simulink model "digitaler_zr"  (R2022b)
settings: Solver=ode45  StartTime=0.0  StopTime=tsim  FixedStep=0.00025  RelTol=1e-3  EnableMultiTasking=on
values from neighbouring files (symbols this model uses):
  A = double(subs(A))    [init1.m]
  B = double(subs(B))    [init1.m]
  C = double(subs(C))    [init1.m]
  q1z = double(subs(q1z))    [init1.m]
  q1zb = double(subs(q1zb))    [init1.m]
  q1zbin = double(subs(q1zbin))    [init1.m]
  R = double(subs(R))    [init1.m]
  Rb = double(subs(Rb))    [init1.m]
  Rbin = double(subs(Rbin))    [init1.m]
  T = 0.5e-3    (= 0.0005)    [init1.m]
  TR = double(subs(TR))    [init1.m]
  tstep = 0.05    [init1.m]
settings Model: Creator=axel  LastModifiedBy=kraie
settings SolverCC: AlgebraicLoopSolver=TrustRegion
settings DataIOCC: LimitDataPoints=on  SaveFormat=Array  SignalLoggingSaveFormat=ModelDataLogs  ReturnWorkspaceOutputs=off
settings OptimizationCC: ExpressionDepthLimit=2147483647  InitFltsAndDblsToZero=on  LifeSpan=inf
settings DebuggingCC: SaveWithParameterizedLinksMsg=none  UnderspecifiedInitializationDetection=Classic  MergeDetectMultiDrivingBlocksExec=none  SignalResolutionControl=TryResolveAllWithWarning  SolverPrmCheckMsg=warning  MultiTaskDSMMsg=warning  MultiTaskCondExecSysMsg=none  FcnCallInpInsideContextMsg=warning  UnconnectedInputMsg=warning  UnconnectedOutputMsg=warning  UnconnectedLineMsg=warning  StateNameClashWarn=warning  SFUnexpectedBacktrackingDiag=warning  SFNoUnconditionalDefaultTransitionDiag=warning  SFMachineParentedDataDiag=warning  ArithmeticOperatorsInVariantConditions=warning
settings HardwareCC: ProdBitPerPointer=32  ProdBitPerSizeT=32  ProdBitPerPtrDiffT=32  ProdLargestAtomicFloat=None  ProdIntDivRoundTo=Undefined  ProdEndianess=Unspecified  ProdWordSize=32  ProdHWDeviceType=32-bit Generic
settings ModelReferenceCC: EnableRefExpFcnMdlSchedulingChecks=on  PropagateSignalLabelsOutOfModel=off
settings SFSimCC: SimUseLocalCustomCode=off  CustomCodeUndefinedFunction=UseInterfaceOnly
settings RTWCC: RTWUseLocalCustomCode=off
settings CodeAppCC: StateflowObjectComments=on
settings GRTTargetCC: TargetFcnLib=ansi_tfl_tmw.mat  TargetLangStandard=C89/C90 (ANSI)  CombineOutputUpdateFcns=off  GRTInterface=on
settings ConfigComp: CovMetricSettings=dw  CovSaveCumulativeToWorkspaceVar=on  CovSaveSingleToWorkspaceVar=on  CovExternalEMLEnable=off

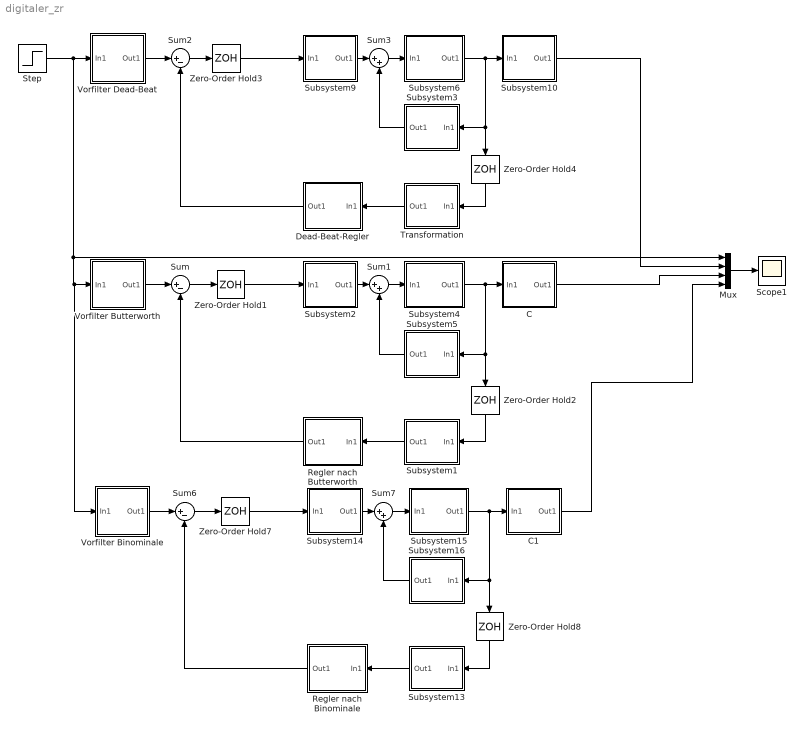
== system digitaler_zr ==
  C : Subsystem
      mask Display: disp('C')
  C1 : Subsystem
      mask Display: disp('C')
  Dead-Beat-Regler : Subsystem
      mask Display: disp('R\nDead-Beat')
  Mux : Mux
  Regler nach Binominale : Subsystem
      mask Display: disp('Rb\nButterworth')
  Regler nach Butterworth : Subsystem
      mask Display: disp('Rb\nButterworth')
  Scope1 : Scope
  Step : Step  Time=tstep  SampleTime=0
  Subsystem1 : Subsystem
      mask Display: disp('TR')
  Subsystem10 : Subsystem
      mask Display: disp('C')
  Subsystem13 : Subsystem
      mask Display: disp('TR')
  Subsystem14 : Subsystem
      mask Display: disp('B')
  Subsystem15 : Subsystem
      mask Display: plot([0.3 0.35 0.4 0.45 0.55 0.6 0.65 0.7], [0.3 0.21 0.2 0.3 0.7 0.8 0.79 0.7]);
  Subsystem16 : Subsystem
      mask Display: disp('A')
  Subsystem2 : Subsystem
      mask Display: disp('B')
  Subsystem3 : Subsystem
      mask Display: disp('A')
  Subsystem4 : Subsystem
      mask Display: plot([0.3 0.35 0.4 0.45 0.55 0.6 0.65 0.7], [0.3 0.21 0.2 0.3 0.7 0.8 0.79 0.7]);
  Subsystem5 : Subsystem
      mask Display: disp('A')
  Subsystem6 : Subsystem
      mask Display: plot([0.3 0.35 0.4 0.45 0.55 0.6 0.65 0.7], [0.3 0.21 0.2 0.3 0.7 0.8 0.79 0.7]);
  Subsystem9 : Subsystem
      mask Display: disp('B')
  Sum : Sum  Inputs=|+-
  Sum1 : Sum  Inputs=|++
  Sum2 : Sum  Inputs=|+-
  Sum3 : Sum  Inputs=|++
  Sum6 : Sum  Inputs=|+-
  Sum7 : Sum  Inputs=|++
  Transformation : Subsystem
      mask Display: disp('TR')
  Vorfilter Binominale : Subsystem
      mask Display: disp('q1zb')
  Vorfilter Butterworth : Subsystem
      mask Display: disp('q1zb')
  Vorfilter Dead-Beat : Subsystem
      mask Display: disp('q1z')
  Zero-Order Hold{1..4,7..8} (6 alike) : ZeroOrderHold  SampleTime=T
  wires:
  Subsystem2/1(Out1) -> Sum1/1
  Sum1/1 -> Subsystem4/1(In1)
  Subsystem5/1(Out1) -> Sum1/2
  Regler nach Butterworth/1(Out1) -> Sum/2
  Subsystem1/1(Out1) -> Regler nach Butterworth/1(In1)
  Sum/1 -> Zero-Order Hold1/1
  Zero-Order Hold2/1 -> Subsystem1/1(In1)
  Vorfilter Butterworth/1(Out1) -> Sum/1
  Subsystem4/1(Out1) -> C/1(In1), Subsystem5/1(In1), Zero-Order Hold2/1
  Subsystem9/1(Out1) -> Sum3/1
  Sum3/1 -> Subsystem6/1(In1)
  Subsystem3/1(Out1) -> Sum3/2
  Dead-Beat-Regler/1(Out1) -> Sum2/2
  Transformation/1(Out1) -> Dead-Beat-Regler/1(In1)
  Sum2/1 -> Zero-Order Hold3/1
  Zero-Order Hold4/1 -> Transformation/1(In1)
  Vorfilter Dead-Beat/1(Out1) -> Sum2/1
  Subsystem6/1(Out1) -> Zero-Order Hold4/1, Subsystem3/1(In1), Subsystem10/1(In1)
  Mux/1 -> Scope1/1
  Zero-Order Hold3/1 -> Subsystem9/1(In1)
  Zero-Order Hold1/1 -> Subsystem2/1(In1)
  Subsystem16/1(Out1) -> Sum7/2
  Sum6/1 -> Zero-Order Hold7/1
  Zero-Order Hold7/1 -> Subsystem14/1(In1)
  Sum7/1 -> Subsystem15/1(In1)
  Regler nach Binominale/1(Out1) -> Sum6/2
  Subsystem13/1(Out1) -> Regler nach Binominale/1(In1)
  Vorfilter Binominale/1(Out1) -> Sum6/1
  Subsystem14/1(Out1) -> Sum7/1
  Subsystem15/1(Out1) -> C1/1(In1), Subsystem16/1(In1), Zero-Order Hold8/1
  Step/1 -> Vorfilter Dead-Beat/1(In1), Mux/1, Vorfilter Binominale/1(In1), Vorfilter Butterworth/1(In1)
  Zero-Order Hold8/1 -> Subsystem13/1(In1)
  C1/1(Out1) -> Mux/4
  Subsystem10/1(Out1) -> Mux/2
  C/1(Out1) -> Mux/3

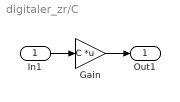
== system digitaler_zr/C ==
  In1 : Inport
  Gain : Gain  Gain=C  Multiplication=Matrix(K*u) (u vector)
  Out1 : Outport
  wires:
  Gain/1 -> Out1/1
  In1/1 -> Gain/1

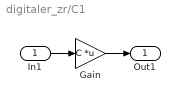
== system digitaler_zr/C1 ==
  In1 : Inport
  Gain : Gain  Gain=C  Multiplication=Matrix(K*u) (u vector)
  Out1 : Outport
  wires:
  Gain/1 -> Out1/1
  In1/1 -> Gain/1

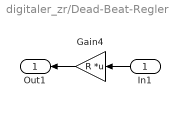
== system digitaler_zr/Dead-Beat-Regler ==
  In1 : Inport
  Gain4 : Gain  Gain=R  Multiplication=Matrix(K*u) (u vector)
  Out1 : Outport
  wires:
  Gain4/1 -> Out1/1
  In1/1 -> Gain4/1

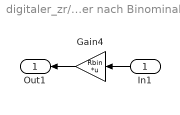
== system digitaler_zr/Regler nach Binominale ==
  In1 : Inport
  Gain4 : Gain  Gain=Rbin  Multiplication=Matrix(K*u) (u vector)
  Out1 : Outport
  wires:
  In1/1 -> Gain4/1
  Gain4/1 -> Out1/1

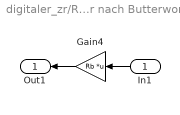
== system digitaler_zr/Regler nach Butterworth ==
  In1 : Inport
  Gain4 : Gain  Gain=Rb  Multiplication=Matrix(K*u) (u vector)
  Out1 : Outport
  wires:
  In1/1 -> Gain4/1
  Gain4/1 -> Out1/1

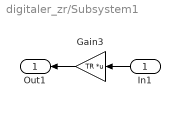
== system digitaler_zr/Subsystem1 ==
  In1 : Inport
  Gain3 : Gain  Gain=TR  Multiplication=Matrix(K*u) (u vector)
  Out1 : Outport
  wires:
  In1/1 -> Gain3/1
  Gain3/1 -> Out1/1

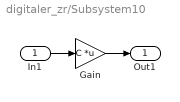
== system digitaler_zr/Subsystem10 ==
  In1 : Inport
  Gain : Gain  Gain=C  Multiplication=Matrix(K*u) (u vector)
  Out1 : Outport
  wires:
  In1/1 -> Gain/1
  Gain/1 -> Out1/1

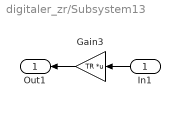
== system digitaler_zr/Subsystem13 ==
  In1 : Inport
  Gain3 : Gain  Gain=TR  Multiplication=Matrix(K*u) (u vector)
  Out1 : Outport
  wires:
  In1/1 -> Gain3/1
  Gain3/1 -> Out1/1

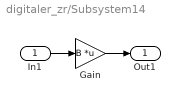
== system digitaler_zr/Subsystem14 ==
  In1 : Inport
  Gain : Gain  Gain=B  Multiplication=Matrix(K*u) (u vector)
  Out1 : Outport
  wires:
  In1/1 -> Gain/1
  Gain/1 -> Out1/1

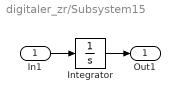
== system digitaler_zr/Subsystem15 ==
  In1 : Inport
  Integrator : Integrator
  Out1 : Outport
  wires:
  In1/1 -> Integrator/1
  Integrator/1 -> Out1/1

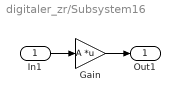
== system digitaler_zr/Subsystem16 ==
  In1 : Inport
  Gain : Gain  Gain=A  Multiplication=Matrix(K*u) (u vector)
  Out1 : Outport
  wires:
  Gain/1 -> Out1/1
  In1/1 -> Gain/1

== system digitaler_zr/Subsystem2 ==
  In1 : Inport
  Gain : Gain  Gain=B  Multiplication=Matrix(K*u) (u vector)
  Out1 : Outport
  wires:
  In1/1 -> Gain/1
  Gain/1 -> Out1/1

== system digitaler_zr/Subsystem3 ==
  In1 : Inport
  Gain : Gain  Gain=A  Multiplication=Matrix(K*u) (u vector)
  Out1 : Outport
  wires:
  In1/1 -> Gain/1
  Gain/1 -> Out1/1

== system digitaler_zr/Subsystem4 ==
  In1 : Inport
  Integrator : Integrator
  Out1 : Outport
  wires:
  In1/1 -> Integrator/1
  Integrator/1 -> Out1/1

== system digitaler_zr/Subsystem5 ==
  In1 : Inport
  Gain : Gain  Gain=A  Multiplication=Matrix(K*u) (u vector)
  Out1 : Outport
  wires:
  Gain/1 -> Out1/1
  In1/1 -> Gain/1

== system digitaler_zr/Subsystem6 ==
  In1 : Inport
  Integrator : Integrator
  Out1 : Outport
  wires:
  Integrator/1 -> Out1/1
  In1/1 -> Integrator/1

== system digitaler_zr/Subsystem9 ==
  In1 : Inport
  Gain : Gain  Gain=B  Multiplication=Matrix(K*u) (u vector)
  Out1 : Outport
  wires:
  Gain/1 -> Out1/1
  In1/1 -> Gain/1

== system digitaler_zr/Transformation ==
  In1 : Inport
  Gain3 : Gain  Gain=TR  Multiplication=Matrix(K*u) (u vector)
  Out1 : Outport
  wires:
  Gain3/1 -> Out1/1
  In1/1 -> Gain3/1

== system digitaler_zr/Vorfilter Binominale ==
  In1 : Inport
  Gain5 : Gain  Gain=q1zbin
  Out1 : Outport
  wires:
  In1/1 -> Gain5/1
  Gain5/1 -> Out1/1

== system digitaler_zr/Vorfilter Butterworth ==
  In1 : Inport
  Gain5 : Gain  Gain=q1zb
  Out1 : Outport
  wires:
  In1/1 -> Gain5/1
  Gain5/1 -> Out1/1

== system digitaler_zr/Vorfilter Dead-Beat ==
  In1 : Inport
  Gain5 : Gain  Gain=q1z
  Out1 : Outport
  wires:
  Gain5/1 -> Out1/1
  In1/1 -> Gain5/1
